simulink model "myfilterbank"  (Simulink 4.00)
settings: Solver=ode45  StartTime=0.0  StopTime=20000  RelTol=1e-3
libraries: ALTELINK x209, simulink_extras x2
settings Model: LastModifiedBy=Administrator

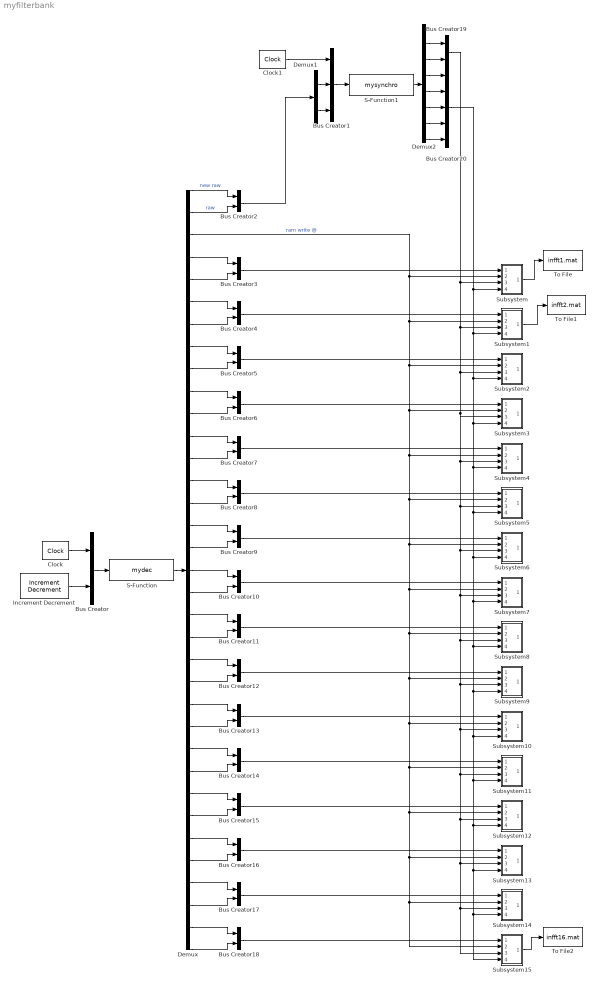
== system myfilterbank ==
  Bus Creator{,2..19} (19 alike) : BusCreator  Inputs=2
  Bus Creator1 : BusCreator  Inputs=3
  Bus Creator20 : BusCreator  Inputs=5
  Clock : simulink_extras/Flip Flops/Clock  MaskParam1=1
  Clock1 : simulink_extras/Flip Flops/Clock  MaskParam1=1
  Demux : Demux  Outputs=35  BusSelectionMode=off
  Demux1 : Demux  Outputs=2  BusSelectionMode=off
  Demux2 : Demux  Outputs=8  BusSelectionMode=off
  Increment Decrement : ALTELINK/Arithmetic/Increment Decrement  BusType=Unsigned Integer  bwl=20  bwr=0  direction=Increment  cst=1  clken=off  MaskValue=1
  S-Function : S-Function  FunctionName=mydec  Parameters=1,256,16,16  PortCounts=[]  SFunctionModules=''
  S-Function1 : S-Function  FunctionName=mysynchro  Parameters=1,256,16,16  PortCounts=[]  SFunctionModules=''
  Subsystem : Subsystem
      settings: RTWFcnNameOpts=Auto  RTWFileNameOpts=Auto
  Subsystem1 : Subsystem
      settings: RTWFcnNameOpts=Auto  RTWFileNameOpts=Auto
  Subsystem10 : Subsystem
      settings: RTWFcnNameOpts=Auto  RTWFileNameOpts=Auto
  Subsystem11 : Subsystem
      settings: RTWFcnNameOpts=Auto  RTWFileNameOpts=Auto
  Subsystem12 : Subsystem
      settings: RTWFcnNameOpts=Auto  RTWFileNameOpts=Auto
  Subsystem13 : Subsystem
      settings: RTWFcnNameOpts=Auto  RTWFileNameOpts=Auto
  Subsystem14 : Subsystem
      settings: RTWFcnNameOpts=Auto  RTWFileNameOpts=Auto
  Subsystem15 : Subsystem
      settings: RTWFcnNameOpts=Auto  RTWFileNameOpts=Auto
  Subsystem2 : Subsystem
      settings: RTWFcnNameOpts=Auto  RTWFileNameOpts=Auto
  Subsystem3 : Subsystem
      settings: RTWFcnNameOpts=Auto  RTWFileNameOpts=Auto
  Subsystem4 : Subsystem
      settings: RTWFcnNameOpts=Auto  RTWFileNameOpts=Auto
  Subsystem5 : Subsystem
      settings: RTWFcnNameOpts=Auto  RTWFileNameOpts=Auto
  Subsystem6 : Subsystem
      settings: RTWFcnNameOpts=Auto  RTWFileNameOpts=Auto
  Subsystem7 : Subsystem
      settings: RTWFcnNameOpts=Auto  RTWFileNameOpts=Auto
  Subsystem8 : Subsystem
      settings: RTWFcnNameOpts=Auto  RTWFileNameOpts=Auto
  Subsystem9 : Subsystem
      settings: RTWFcnNameOpts=Auto  RTWFileNameOpts=Auto
  To File : ToFile  Filename=infft1.mat  MatrixName=sig1  SampleTime=-1
  To File1 : ToFile  Filename=infft2.mat  MatrixName=sig2  SampleTime=-1
  To File2 : ToFile  Filename=infft16.mat  MatrixName=sig16  SampleTime=-1
  wires:
  S-Function/1 -> Demux/1
  Bus Creator/1 -> S-Function/1
  Clock/1 -> Bus Creator/1
  Increment Decrement/1 -> Bus Creator/2
  Demux/3 -> Subsystem/2(In2), Subsystem1/2(In2), Subsystem2/2(In2), Subsystem3/2(In2), Subsystem4/2(In2), Subsystem5/2(In2), Subsystem6/2(In2), Subsystem7/2(In2), Subsystem8/2(In2), Subsystem9/2(In2), Subsystem10/2(In2), Subsystem11/2(In2), Subsystem12/2(In2), Subsystem13/2(In2), Subsystem14/2(In2), Subsystem15/2(In2)  "ram write @"
  Clock1/1 -> Bus Creator1/1
  Bus Creator1/1 -> S-Function1/1
  Demux/1 -> Bus Creator2/1  "new raw"
  Demux/2 -> Bus Creator2/2  "raw"
  Bus Creator2/1 -> Demux1/1
  Demux1/1 -> Bus Creator1/2
  Demux1/2 -> Bus Creator1/3
  Demux/4 -> Bus Creator3/1
  Demux/5 -> Bus Creator3/2
  Bus Creator3/1 -> Subsystem/1(In1)
  Demux/6 -> Bus Creator4/1
  Demux/7 -> Bus Creator4/2
  Demux/8 -> Bus Creator5/1
  Demux/9 -> Bus Creator5/2
  Demux/10 -> Bus Creator6/1
  Demux/11 -> Bus Creator6/2
  Demux/12 -> Bus Creator7/1
  Demux/13 -> Bus Creator7/2
  Demux/14 -> Bus Creator8/1
  Demux/15 -> Bus Creator8/2
  Demux/16 -> Bus Creator9/1
  Demux/17 -> Bus Creator9/2
  Demux/18 -> Bus Creator10/1
  Demux/19 -> Bus Creator10/2
  Demux/20 -> Bus Creator11/1
  Demux/21 -> Bus Creator11/2
  Demux/22 -> Bus Creator12/1
  Demux/23 -> Bus Creator12/2
  Demux/24 -> Bus Creator13/1
  Demux/25 -> Bus Creator13/2
  Demux/26 -> Bus Creator14/1
  Demux/27 -> Bus Creator14/2
  Demux/28 -> Bus Creator15/1
  Demux/29 -> Bus Creator15/2
  Demux/30 -> Bus Creator16/1
  Demux/31 -> Bus Creator16/2
  Demux/32 -> Bus Creator17/1
  Demux/33 -> Bus Creator17/2
  Demux/34 -> Bus Creator18/1
  Demux/35 -> Bus Creator18/2
  Demux2/3 -> Bus Creator19/2
  Demux2/2 -> Bus Creator19/1
  Bus Creator19/1 -> Subsystem/3(In3), Subsystem1/3(In3), Subsystem2/3(In3), Subsystem3/3(In3), Subsystem4/3(In3), Subsystem5/3(In3), Subsystem6/3(In3), Subsystem7/3(In3), Subsystem8/3(In3), Subsystem9/3(In3), Subsystem10/3(In3), Subsystem11/3(In3), Subsystem12/3(In3), Subsystem13/3(In3), Subsystem14/3(In3), Subsystem15/3(In3)
  S-Function1/1 -> Demux2/1
  Demux2/4 -> Bus Creator20/1
  Demux2/5 -> Bus Creator20/2
  Demux2/6 -> Bus Creator20/3
  Demux2/7 -> Bus Creator20/4
  Demux2/8 -> Bus Creator20/5
  Bus Creator20/1 -> Subsystem/4(In4), Subsystem1/4(In4), Subsystem2/4(In4), Subsystem3/4(In4), Subsystem4/4(In4), Subsystem5/4(In4), Subsystem6/4(In4), Subsystem7/4(In4), Subsystem8/4(In4), Subsystem9/4(In4), Subsystem10/4(In4), Subsystem11/4(In4), Subsystem12/4(In4), Subsystem13/4(In4), Subsystem14/4(In4), Subsystem15/4(In4)
  Subsystem/1(Out1) -> To File/1
  Bus Creator4/1 -> Subsystem1/1(In1)
  Bus Creator5/1 -> Subsystem2/1(In1)
  Bus Creator6/1 -> Subsystem3/1(In1)
  Subsystem1/1(Out1) -> To File1/1
  Bus Creator7/1 -> Subsystem4/1(In1)
  Bus Creator8/1 -> Subsystem5/1(In1)
  Bus Creator9/1 -> Subsystem6/1(In1)
  Bus Creator10/1 -> Subsystem7/1(In1)
  Bus Creator11/1 -> Subsystem8/1(In1)
  Bus Creator12/1 -> Subsystem9/1(In1)
  Bus Creator13/1 -> Subsystem10/1(In1)
  Bus Creator14/1 -> Subsystem11/1(In1)
  Bus Creator15/1 -> Subsystem12/1(In1)
  Bus Creator16/1 -> Subsystem13/1(In1)
  Bus Creator17/1 -> Subsystem14/1(In1)
  Bus Creator18/1 -> Subsystem15/1(In1)
  Subsystem15/1(Out1) -> To File2/1

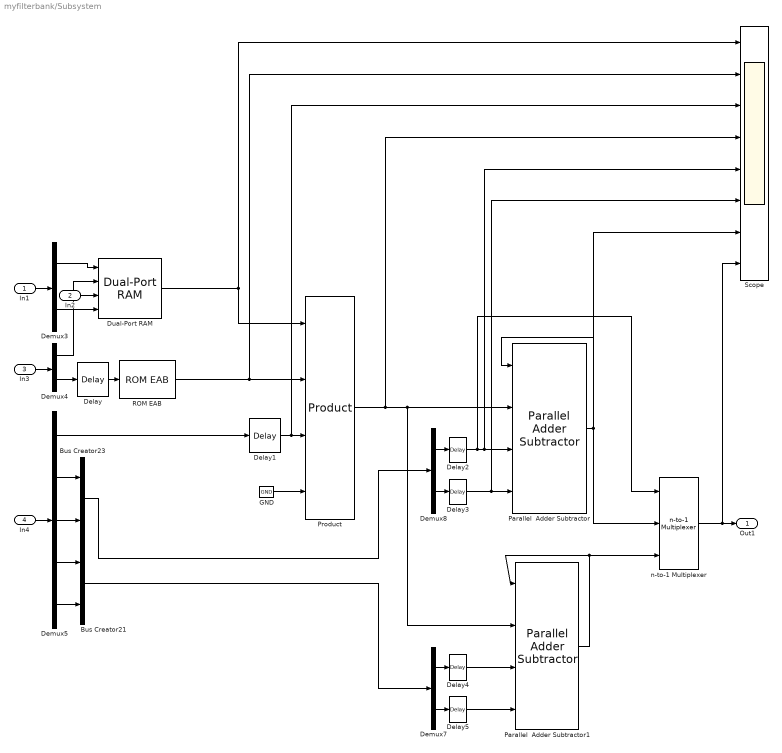
== system myfilterbank/Subsystem ==
  In1 : Inport  Port=1  LatchInput=off
  In2 : Inport  Port=2  LatchInput=off
  In3 : Inport  Port=3  LatchInput=off
  In4 : Inport  Port=4  LatchInput=off
  Bus Creator21 : BusCreator  Inputs=2
  Bus Creator23 : BusCreator  Inputs=2
  Delay : ALTELINK/Storage/Delay  depth=1  clken=off  MaskValue=1
  Delay1 : ALTELINK/Storage/Delay  depth=2  clken=off  MaskValue=1
  Delay{2..5} (4 alike) : ALTELINK/Storage/Delay  depth=3  clken=off  MaskValue=1
  Demux{3..4,7..8} (4 alike) : Demux  Outputs=2  BusSelectionMode=off
  Demux5 : Demux  Outputs=5  BusSelectionMode=off
  Dual-Port RAM : ALTELINK/Storage/Dual-Port RAM  bwaddr=9  MaskValue=1
  GND : ALTELINK/Bus Manipulation/GND
  Parallel  Adder Subtractor : ALTELINK/Arithmetic/Parallel  Adder Subtractor  Inputs=2  direction=++  pipeline=on  clken=on  MaskValue=1
  Parallel  Adder Subtractor1 : ALTELINK/Arithmetic/Parallel  Adder Subtractor  Inputs=2  direction=++  pipeline=on  clken=on  MaskValue=1
  Product : ALTELINK/Arithmetic/Product  pipeline=1  lpm=off  eab=off  clken=on  MaskValue=1
  ROM EAB : ALTELINK/Storage/ROM EAB  BusType=Signed Integer  bwl=14  bwr=0  bwaddr=8  Inputs=sub1.hex  MaskValue=1
  Scope : Scope  NumInputPorts=8
      settings: TimeRange=106.7708333333333  YMin=-5~-5~-5~-5~-5~0~-5~-5  YMax=5~5~5~5~5~1~5~5  SaveToWorkspace=off  SaveName=ScopeData  LimitDataPoints=on  MaxDataPoints=20000
  n-to-1 Multiplexer : ALTELINK/Gates/n-to-1 Multiplexer  Inputs=2  BusType=off
  Out1 : Outport  Port=1
  wires:
  Dual-Port RAM/1 -> Product/1, Scope/1
  ROM EAB/1 -> Product/2, Scope/2
  Product/1 -> Parallel  Adder Subtractor/2, Parallel  Adder Subtractor1/2, Scope/4
  Parallel  Adder Subtractor1/1 -> Parallel  Adder Subtractor1/1, n-to-1 Multiplexer/3
  Parallel  Adder Subtractor/1 -> Parallel  Adder Subtractor/1, Scope/7, n-to-1 Multiplexer/2
  Delay/1 -> ROM EAB/1
  GND/1 -> Product/4
  Demux3/2 -> Dual-Port RAM/4
  Demux3/1 -> Dual-Port RAM/1
  Demux4/1 -> Dual-Port RAM/2
  Demux4/2 -> Delay/1
  Demux5/1 -> Delay1/1
  Delay1/1 -> Product/3, Scope/3
  Demux7/2 -> Delay5/1
  Demux7/1 -> Delay4/1
  Demux8/2 -> Delay3/1
  Demux8/1 -> Delay2/1
  Demux5/5 -> Bus Creator21/2
  Demux5/4 -> Bus Creator21/1
  Demux5/3 -> Bus Creator23/2
  Demux5/2 -> Bus Creator23/1
  Bus Creator21/1 -> Demux7/1
  Bus Creator23/1 -> Demux8/1
  Delay2/1 -> n-to-1 Multiplexer/1, Parallel  Adder Subtractor/3, Scope/5
  Delay3/1 -> Parallel  Adder Subtractor/4, Scope/6
  Delay4/1 -> Parallel  Adder Subtractor1/3
  Delay5/1 -> Parallel  Adder Subtractor1/4
  n-to-1 Multiplexer/1 -> Scope/8, Out1/1
  In1/1 -> Demux3/1
  In2/1 -> Dual-Port RAM/3
  In3/1 -> Demux4/1
  In4/1 -> Demux5/1

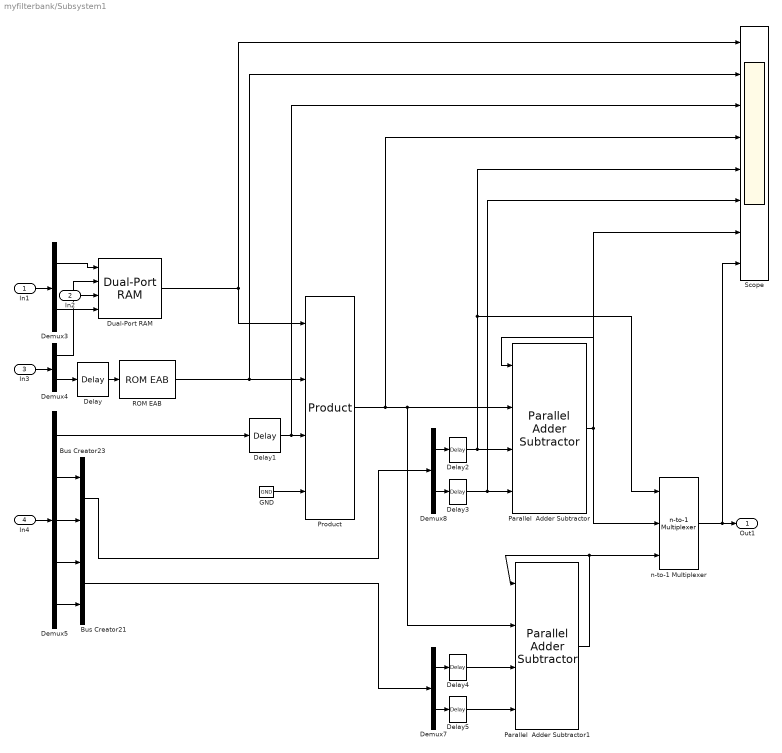
== system myfilterbank/Subsystem1 ==
  In1 : Inport  Port=1  LatchInput=off
  In2 : Inport  Port=2  LatchInput=off
  In3 : Inport  Port=3  LatchInput=off
  In4 : Inport  Port=4  LatchInput=off
  Bus Creator21 : BusCreator  Inputs=2
  Bus Creator23 : BusCreator  Inputs=2
  Delay : ALTELINK/Storage/Delay  depth=1  clken=off  MaskValue=1
  Delay1 : ALTELINK/Storage/Delay  depth=2  clken=off  MaskValue=1
  Delay{2..5} (4 alike) : ALTELINK/Storage/Delay  depth=3  clken=off  MaskValue=1
  Demux{3..4,7..8} (4 alike) : Demux  Outputs=2  BusSelectionMode=off
  Demux5 : Demux  Outputs=5  BusSelectionMode=off
  Dual-Port RAM : ALTELINK/Storage/Dual-Port RAM  bwaddr=9  MaskValue=1
  GND : ALTELINK/Bus Manipulation/GND
  Parallel  Adder Subtractor : ALTELINK/Arithmetic/Parallel  Adder Subtractor  Inputs=2  direction=++  pipeline=on  clken=on  MaskValue=1
  Parallel  Adder Subtractor1 : ALTELINK/Arithmetic/Parallel  Adder Subtractor  Inputs=2  direction=++  pipeline=on  clken=on  MaskValue=1
  Product : ALTELINK/Arithmetic/Product  pipeline=1  lpm=off  eab=off  clken=on  MaskValue=1
  ROM EAB : ALTELINK/Storage/ROM EAB  BusType=Signed Integer  bwl=14  bwr=0  bwaddr=9  Inputs=onlyone.hex  MaskValue=1
  Scope : Scope  NumInputPorts=8
      settings: TimeRange=auto  YMin=-5~-5~-5~-5~-5~-5~-5~-5  YMax=5~5~5~5~5~5~5~5  SaveToWorkspace=off  SaveName=ScopeData  LimitDataPoints=on  MaxDataPoints=20000
  n-to-1 Multiplexer : ALTELINK/Gates/n-to-1 Multiplexer  Inputs=2  BusType=off
  Out1 : Outport  Port=1
  wires:
  Dual-Port RAM/1 -> Product/1, Scope/1
  ROM EAB/1 -> Product/2, Scope/2
  Product/1 -> Parallel  Adder Subtractor/2, Parallel  Adder Subtractor1/2, Scope/4
  Parallel  Adder Subtractor1/1 -> Parallel  Adder Subtractor1/1, n-to-1 Multiplexer/3
  Parallel  Adder Subtractor/1 -> Parallel  Adder Subtractor/1, Scope/7, n-to-1 Multiplexer/2
  Delay/1 -> ROM EAB/1
  GND/1 -> Product/4
  Demux3/2 -> Dual-Port RAM/4
  Demux3/1 -> Dual-Port RAM/1
  Demux4/1 -> Dual-Port RAM/2
  Demux4/2 -> Delay/1
  Demux5/1 -> Delay1/1
  Delay1/1 -> Product/3, Scope/3
  Demux7/2 -> Delay5/1
  Demux7/1 -> Delay4/1
  Demux8/2 -> Delay3/1
  Demux8/1 -> Delay2/1
  Demux5/5 -> Bus Creator21/2
  Demux5/4 -> Bus Creator21/1
  Demux5/3 -> Bus Creator23/2
  Demux5/2 -> Bus Creator23/1
  Bus Creator21/1 -> Demux7/1
  Bus Creator23/1 -> Demux8/1
  Delay2/1 -> Parallel  Adder Subtractor/3, Scope/5, n-to-1 Multiplexer/1
  Delay3/1 -> Parallel  Adder Subtractor/4, Scope/6
  Delay4/1 -> Parallel  Adder Subtractor1/3
  Delay5/1 -> Parallel  Adder Subtractor1/4
  n-to-1 Multiplexer/1 -> Scope/8, Out1/1
  In1/1 -> Demux3/1
  In2/1 -> Dual-Port RAM/3
  In3/1 -> Demux4/1
  In4/1 -> Demux5/1

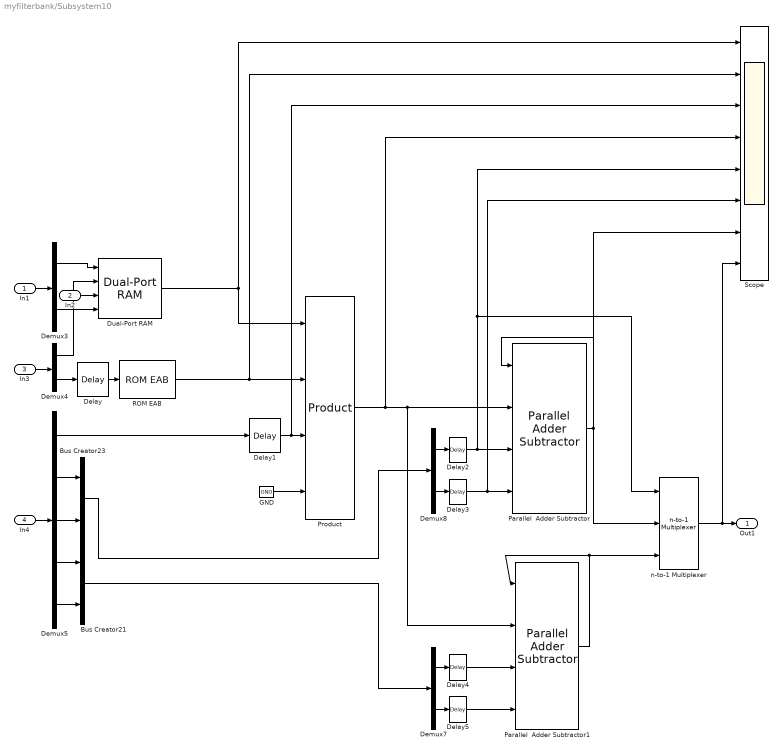
== system myfilterbank/Subsystem10 ==
  In1 : Inport  Port=1  LatchInput=off
  In2 : Inport  Port=2  LatchInput=off
  In3 : Inport  Port=3  LatchInput=off
  In4 : Inport  Port=4  LatchInput=off
  Bus Creator21 : BusCreator  Inputs=2
  Bus Creator23 : BusCreator  Inputs=2
  Delay : ALTELINK/Storage/Delay  depth=1  clken=off  MaskValue=1
  Delay1 : ALTELINK/Storage/Delay  depth=2  clken=off  MaskValue=1
  Delay{2..5} (4 alike) : ALTELINK/Storage/Delay  depth=3  clken=off  MaskValue=1
  Demux{3..4,7..8} (4 alike) : Demux  Outputs=2  BusSelectionMode=off
  Demux5 : Demux  Outputs=5  BusSelectionMode=off
  Dual-Port RAM : ALTELINK/Storage/Dual-Port RAM  bwaddr=9  MaskValue=1
  GND : ALTELINK/Bus Manipulation/GND
  Parallel  Adder Subtractor : ALTELINK/Arithmetic/Parallel  Adder Subtractor  Inputs=2  direction=++  pipeline=on  clken=on  MaskValue=1
  Parallel  Adder Subtractor1 : ALTELINK/Arithmetic/Parallel  Adder Subtractor  Inputs=2  direction=++  pipeline=on  clken=on  MaskValue=1
  Product : ALTELINK/Arithmetic/Product  pipeline=1  lpm=off  eab=off  clken=on  MaskValue=1
  ROM EAB : ALTELINK/Storage/ROM EAB  BusType=Signed Integer  bwl=14  bwr=0  bwaddr=9  Inputs=onlyone.hex  MaskValue=1
  Scope : Scope  NumInputPorts=8
      settings: TimeRange=auto  YMin=-5~-5~-5~-5~-5~-5~-5~-5  YMax=5~5~5~5~5~5~5~5  SaveToWorkspace=off  SaveName=ScopeData  LimitDataPoints=on  MaxDataPoints=20000
  n-to-1 Multiplexer : ALTELINK/Gates/n-to-1 Multiplexer  Inputs=2  BusType=off
  Out1 : Outport  Port=1
  wires:
  Dual-Port RAM/1 -> Product/1, Scope/1
  ROM EAB/1 -> Product/2, Scope/2
  Product/1 -> Parallel  Adder Subtractor/2, Parallel  Adder Subtractor1/2, Scope/4
  Parallel  Adder Subtractor1/1 -> Parallel  Adder Subtractor1/1, n-to-1 Multiplexer/3
  Parallel  Adder Subtractor/1 -> Parallel  Adder Subtractor/1, Scope/7, n-to-1 Multiplexer/2
  Delay/1 -> ROM EAB/1
  GND/1 -> Product/4
  Demux3/2 -> Dual-Port RAM/4
  Demux3/1 -> Dual-Port RAM/1
  Demux4/1 -> Dual-Port RAM/2
  Demux4/2 -> Delay/1
  Demux5/1 -> Delay1/1
  Delay1/1 -> Product/3, Scope/3
  Demux7/2 -> Delay5/1
  Demux7/1 -> Delay4/1
  Demux8/2 -> Delay3/1
  Demux8/1 -> Delay2/1
  Demux5/5 -> Bus Creator21/2
  Demux5/4 -> Bus Creator21/1
  Demux5/3 -> Bus Creator23/2
  Demux5/2 -> Bus Creator23/1
  Bus Creator21/1 -> Demux7/1
  Bus Creator23/1 -> Demux8/1
  Delay2/1 -> Parallel  Adder Subtractor/3, Scope/5, n-to-1 Multiplexer/1
  Delay3/1 -> Parallel  Adder Subtractor/4, Scope/6
  Delay4/1 -> Parallel  Adder Subtractor1/3
  Delay5/1 -> Parallel  Adder Subtractor1/4
  n-to-1 Multiplexer/1 -> Scope/8, Out1/1
  In1/1 -> Demux3/1
  In2/1 -> Dual-Port RAM/3
  In3/1 -> Demux4/1
  In4/1 -> Demux5/1

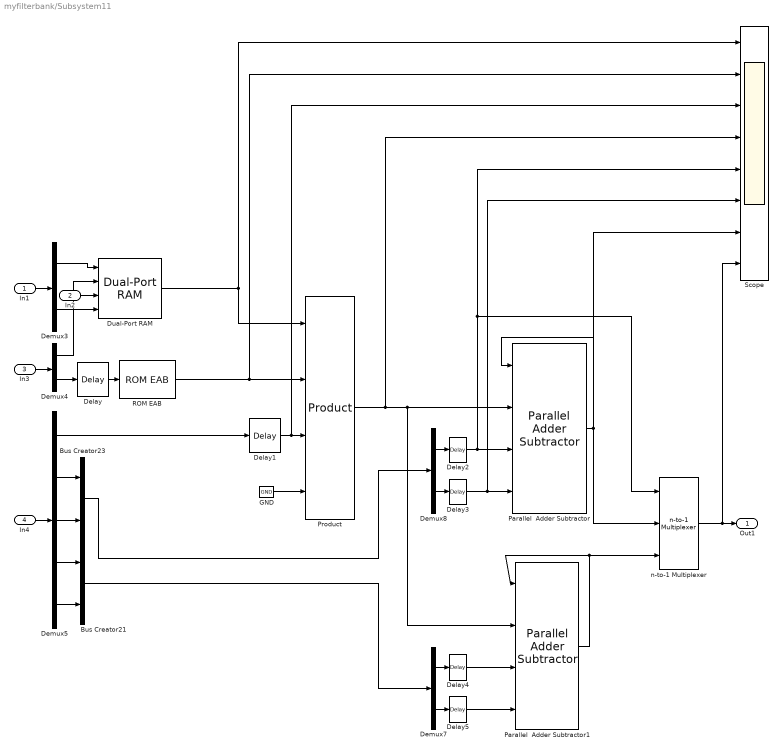
== system myfilterbank/Subsystem11 ==
  In1 : Inport  Port=1  LatchInput=off
  In2 : Inport  Port=2  LatchInput=off
  In3 : Inport  Port=3  LatchInput=off
  In4 : Inport  Port=4  LatchInput=off
  Bus Creator21 : BusCreator  Inputs=2
  Bus Creator23 : BusCreator  Inputs=2
  Delay : ALTELINK/Storage/Delay  depth=1  clken=off  MaskValue=1
  Delay1 : ALTELINK/Storage/Delay  depth=2  clken=off  MaskValue=1
  Delay{2..5} (4 alike) : ALTELINK/Storage/Delay  depth=3  clken=off  MaskValue=1
  Demux{3..4,7..8} (4 alike) : Demux  Outputs=2  BusSelectionMode=off
  Demux5 : Demux  Outputs=5  BusSelectionMode=off
  Dual-Port RAM : ALTELINK/Storage/Dual-Port RAM  bwaddr=9  MaskValue=1
  GND : ALTELINK/Bus Manipulation/GND
  Parallel  Adder Subtractor : ALTELINK/Arithmetic/Parallel  Adder Subtractor  Inputs=2  direction=++  pipeline=on  clken=on  MaskValue=1
  Parallel  Adder Subtractor1 : ALTELINK/Arithmetic/Parallel  Adder Subtractor  Inputs=2  direction=++  pipeline=on  clken=on  MaskValue=1
  Product : ALTELINK/Arithmetic/Product  pipeline=1  lpm=off  eab=off  clken=on  MaskValue=1
  ROM EAB : ALTELINK/Storage/ROM EAB  BusType=Signed Integer  bwl=14  bwr=0  bwaddr=9  Inputs=onlyone.hex  MaskValue=1
  Scope : Scope  NumInputPorts=8
      settings: TimeRange=auto  YMin=-5~-5~-5~-5~-5~-5~-5~-5  YMax=5~5~5~5~5~5~5~5  SaveToWorkspace=off  SaveName=ScopeData  LimitDataPoints=on  MaxDataPoints=20000
  n-to-1 Multiplexer : ALTELINK/Gates/n-to-1 Multiplexer  Inputs=2  BusType=off
  Out1 : Outport  Port=1
  wires:
  Dual-Port RAM/1 -> Product/1, Scope/1
  ROM EAB/1 -> Product/2, Scope/2
  Product/1 -> Parallel  Adder Subtractor/2, Parallel  Adder Subtractor1/2, Scope/4
  Parallel  Adder Subtractor1/1 -> Parallel  Adder Subtractor1/1, n-to-1 Multiplexer/3
  Parallel  Adder Subtractor/1 -> Parallel  Adder Subtractor/1, Scope/7, n-to-1 Multiplexer/2
  Delay/1 -> ROM EAB/1
  GND/1 -> Product/4
  Demux3/2 -> Dual-Port RAM/4
  Demux3/1 -> Dual-Port RAM/1
  Demux4/1 -> Dual-Port RAM/2
  Demux4/2 -> Delay/1
  Demux5/1 -> Delay1/1
  Delay1/1 -> Product/3, Scope/3
  Demux7/2 -> Delay5/1
  Demux7/1 -> Delay4/1
  Demux8/2 -> Delay3/1
  Demux8/1 -> Delay2/1
  Demux5/5 -> Bus Creator21/2
  Demux5/4 -> Bus Creator21/1
  Demux5/3 -> Bus Creator23/2
  Demux5/2 -> Bus Creator23/1
  Bus Creator21/1 -> Demux7/1
  Bus Creator23/1 -> Demux8/1
  Delay2/1 -> Parallel  Adder Subtractor/3, Scope/5, n-to-1 Multiplexer/1
  Delay3/1 -> Parallel  Adder Subtractor/4, Scope/6
  Delay4/1 -> Parallel  Adder Subtractor1/3
  Delay5/1 -> Parallel  Adder Subtractor1/4
  n-to-1 Multiplexer/1 -> Scope/8, Out1/1
  In1/1 -> Demux3/1
  In2/1 -> Dual-Port RAM/3
  In3/1 -> Demux4/1
  In4/1 -> Demux5/1

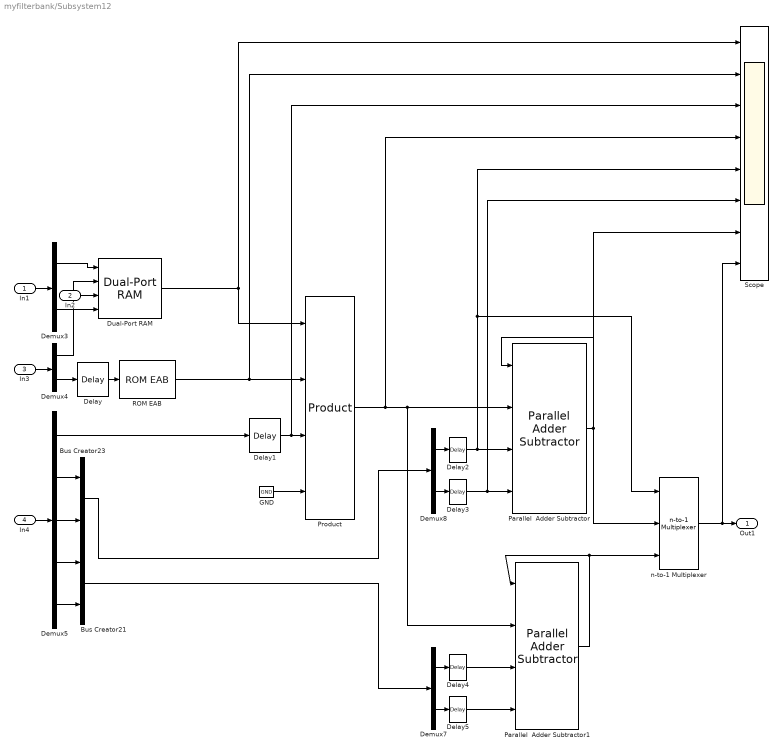
== system myfilterbank/Subsystem12 ==
  In1 : Inport  Port=1  LatchInput=off
  In2 : Inport  Port=2  LatchInput=off
  In3 : Inport  Port=3  LatchInput=off
  In4 : Inport  Port=4  LatchInput=off
  Bus Creator21 : BusCreator  Inputs=2
  Bus Creator23 : BusCreator  Inputs=2
  Delay : ALTELINK/Storage/Delay  depth=1  clken=off  MaskValue=1
  Delay1 : ALTELINK/Storage/Delay  depth=2  clken=off  MaskValue=1
  Delay{2..5} (4 alike) : ALTELINK/Storage/Delay  depth=3  clken=off  MaskValue=1
  Demux{3..4,7..8} (4 alike) : Demux  Outputs=2  BusSelectionMode=off
  Demux5 : Demux  Outputs=5  BusSelectionMode=off
  Dual-Port RAM : ALTELINK/Storage/Dual-Port RAM  bwaddr=9  MaskValue=1
  GND : ALTELINK/Bus Manipulation/GND
  Parallel  Adder Subtractor : ALTELINK/Arithmetic/Parallel  Adder Subtractor  Inputs=2  direction=++  pipeline=on  clken=on  MaskValue=1
  Parallel  Adder Subtractor1 : ALTELINK/Arithmetic/Parallel  Adder Subtractor  Inputs=2  direction=++  pipeline=on  clken=on  MaskValue=1
  Product : ALTELINK/Arithmetic/Product  pipeline=1  lpm=off  eab=off  clken=on  MaskValue=1
  ROM EAB : ALTELINK/Storage/ROM EAB  BusType=Signed Integer  bwl=14  bwr=0  bwaddr=9  Inputs=onlyone.hex  MaskValue=1
  Scope : Scope  NumInputPorts=8
      settings: TimeRange=auto  YMin=-5~-5~-5~-5~-5~-5~-5~-5  YMax=5~5~5~5~5~5~5~5  SaveToWorkspace=off  SaveName=ScopeData  LimitDataPoints=on  MaxDataPoints=20000
  n-to-1 Multiplexer : ALTELINK/Gates/n-to-1 Multiplexer  Inputs=2  BusType=off
  Out1 : Outport  Port=1
  wires:
  Dual-Port RAM/1 -> Product/1, Scope/1
  ROM EAB/1 -> Product/2, Scope/2
  Product/1 -> Parallel  Adder Subtractor/2, Parallel  Adder Subtractor1/2, Scope/4
  Parallel  Adder Subtractor1/1 -> Parallel  Adder Subtractor1/1, n-to-1 Multiplexer/3
  Parallel  Adder Subtractor/1 -> Parallel  Adder Subtractor/1, Scope/7, n-to-1 Multiplexer/2
  Delay/1 -> ROM EAB/1
  GND/1 -> Product/4
  Demux3/2 -> Dual-Port RAM/4
  Demux3/1 -> Dual-Port RAM/1
  Demux4/1 -> Dual-Port RAM/2
  Demux4/2 -> Delay/1
  Demux5/1 -> Delay1/1
  Delay1/1 -> Product/3, Scope/3
  Demux7/2 -> Delay5/1
  Demux7/1 -> Delay4/1
  Demux8/2 -> Delay3/1
  Demux8/1 -> Delay2/1
  Demux5/5 -> Bus Creator21/2
  Demux5/4 -> Bus Creator21/1
  Demux5/3 -> Bus Creator23/2
  Demux5/2 -> Bus Creator23/1
  Bus Creator21/1 -> Demux7/1
  Bus Creator23/1 -> Demux8/1
  Delay2/1 -> Parallel  Adder Subtractor/3, Scope/5, n-to-1 Multiplexer/1
  Delay3/1 -> Parallel  Adder Subtractor/4, Scope/6
  Delay4/1 -> Parallel  Adder Subtractor1/3
  Delay5/1 -> Parallel  Adder Subtractor1/4
  n-to-1 Multiplexer/1 -> Scope/8, Out1/1
  In1/1 -> Demux3/1
  In2/1 -> Dual-Port RAM/3
  In3/1 -> Demux4/1
  In4/1 -> Demux5/1

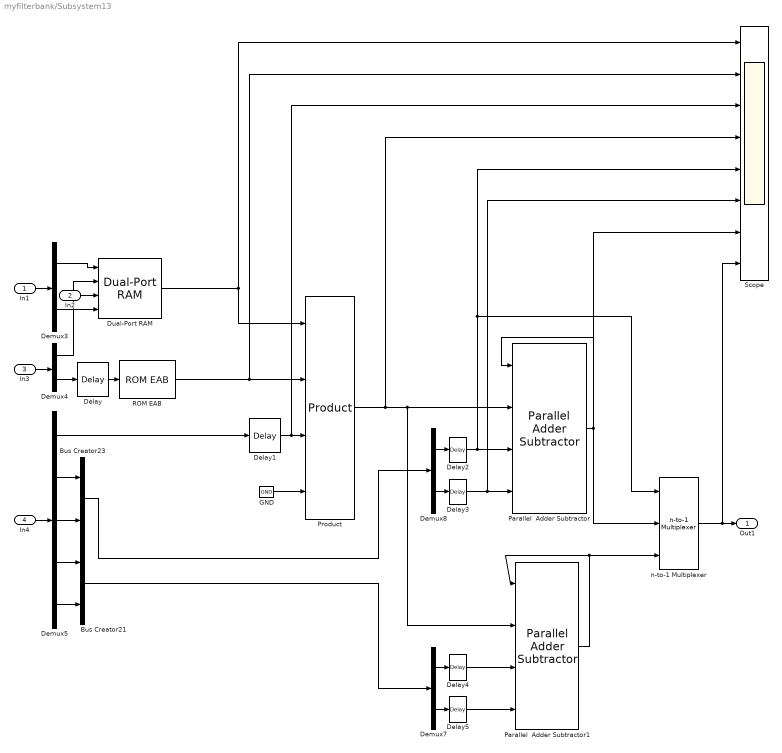
== system myfilterbank/Subsystem13 ==
  In1 : Inport  Port=1  LatchInput=off
  In2 : Inport  Port=2  LatchInput=off
  In3 : Inport  Port=3  LatchInput=off
  In4 : Inport  Port=4  LatchInput=off
  Bus Creator21 : BusCreator  Inputs=2
  Bus Creator23 : BusCreator  Inputs=2
  Delay : ALTELINK/Storage/Delay  depth=1  clken=off  MaskValue=1
  Delay1 : ALTELINK/Storage/Delay  depth=2  clken=off  MaskValue=1
  Delay{2..5} (4 alike) : ALTELINK/Storage/Delay  depth=3  clken=off  MaskValue=1
  Demux{3..4,7..8} (4 alike) : Demux  Outputs=2  BusSelectionMode=off
  Demux5 : Demux  Outputs=5  BusSelectionMode=off
  Dual-Port RAM : ALTELINK/Storage/Dual-Port RAM  bwaddr=9  MaskValue=1
  GND : ALTELINK/Bus Manipulation/GND
  Parallel  Adder Subtractor : ALTELINK/Arithmetic/Parallel  Adder Subtractor  Inputs=2  direction=++  pipeline=on  clken=on  MaskValue=1
  Parallel  Adder Subtractor1 : ALTELINK/Arithmetic/Parallel  Adder Subtractor  Inputs=2  direction=++  pipeline=on  clken=on  MaskValue=1
  Product : ALTELINK/Arithmetic/Product  pipeline=1  lpm=off  eab=off  clken=on  MaskValue=1
  ROM EAB : ALTELINK/Storage/ROM EAB  BusType=Signed Integer  bwl=14  bwr=0  bwaddr=9  Inputs=onlyone.hex  MaskValue=1
  Scope : Scope  NumInputPorts=8
      settings: TimeRange=auto  YMin=-5~-5~-5~-5~-5~-5~-5~-5  YMax=5~5~5~5~5~5~5~5  SaveToWorkspace=off  SaveName=ScopeData  LimitDataPoints=on  MaxDataPoints=20000
  n-to-1 Multiplexer : ALTELINK/Gates/n-to-1 Multiplexer  Inputs=2  BusType=off
  Out1 : Outport  Port=1
  wires:
  Dual-Port RAM/1 -> Product/1, Scope/1
  ROM EAB/1 -> Product/2, Scope/2
  Product/1 -> Parallel  Adder Subtractor/2, Parallel  Adder Subtractor1/2, Scope/4
  Parallel  Adder Subtractor1/1 -> Parallel  Adder Subtractor1/1, n-to-1 Multiplexer/3
  Parallel  Adder Subtractor/1 -> Parallel  Adder Subtractor/1, Scope/7, n-to-1 Multiplexer/2
  Delay/1 -> ROM EAB/1
  GND/1 -> Product/4
  Demux3/2 -> Dual-Port RAM/4
  Demux3/1 -> Dual-Port RAM/1
  Demux4/1 -> Dual-Port RAM/2
  Demux4/2 -> Delay/1
  Demux5/1 -> Delay1/1
  Delay1/1 -> Product/3, Scope/3
  Demux7/2 -> Delay5/1
  Demux7/1 -> Delay4/1
  Demux8/2 -> Delay3/1
  Demux8/1 -> Delay2/1
  Demux5/5 -> Bus Creator21/2
  Demux5/4 -> Bus Creator21/1
  Demux5/3 -> Bus Creator23/2
  Demux5/2 -> Bus Creator23/1
  Bus Creator21/1 -> Demux7/1
  Bus Creator23/1 -> Demux8/1
  Delay2/1 -> Parallel  Adder Subtractor/3, Scope/5, n-to-1 Multiplexer/1
  Delay3/1 -> Parallel  Adder Subtractor/4, Scope/6
  Delay4/1 -> Parallel  Adder Subtractor1/3
  Delay5/1 -> Parallel  Adder Subtractor1/4
  n-to-1 Multiplexer/1 -> Scope/8, Out1/1
  In1/1 -> Demux3/1
  In2/1 -> Dual-Port RAM/3
  In3/1 -> Demux4/1
  In4/1 -> Demux5/1

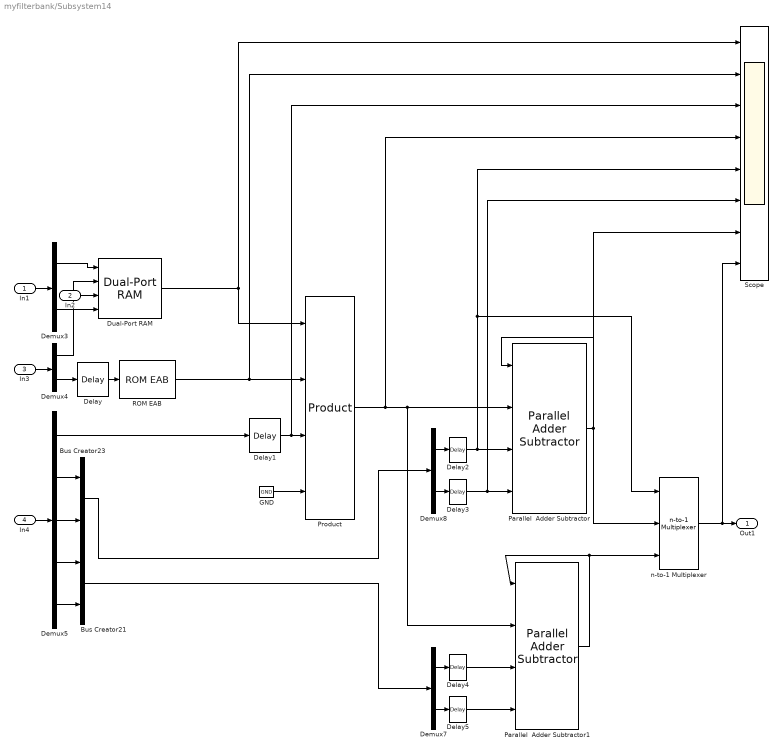
== system myfilterbank/Subsystem14 ==
  In1 : Inport  Port=1  LatchInput=off
  In2 : Inport  Port=2  LatchInput=off
  In3 : Inport  Port=3  LatchInput=off
  In4 : Inport  Port=4  LatchInput=off
  Bus Creator21 : BusCreator  Inputs=2
  Bus Creator23 : BusCreator  Inputs=2
  Delay : ALTELINK/Storage/Delay  depth=1  clken=off  MaskValue=1
  Delay1 : ALTELINK/Storage/Delay  depth=2  clken=off  MaskValue=1
  Delay{2..5} (4 alike) : ALTELINK/Storage/Delay  depth=3  clken=off  MaskValue=1
  Demux{3..4,7..8} (4 alike) : Demux  Outputs=2  BusSelectionMode=off
  Demux5 : Demux  Outputs=5  BusSelectionMode=off
  Dual-Port RAM : ALTELINK/Storage/Dual-Port RAM  bwaddr=9  MaskValue=1
  GND : ALTELINK/Bus Manipulation/GND
  Parallel  Adder Subtractor : ALTELINK/Arithmetic/Parallel  Adder Subtractor  Inputs=2  direction=++  pipeline=on  clken=on  MaskValue=1
  Parallel  Adder Subtractor1 : ALTELINK/Arithmetic/Parallel  Adder Subtractor  Inputs=2  direction=++  pipeline=on  clken=on  MaskValue=1
  Product : ALTELINK/Arithmetic/Product  pipeline=1  lpm=off  eab=off  clken=on  MaskValue=1
  ROM EAB : ALTELINK/Storage/ROM EAB  BusType=Signed Integer  bwl=14  bwr=0  bwaddr=9  Inputs=onlyone.hex  MaskValue=1
  Scope : Scope  NumInputPorts=8
      settings: TimeRange=auto  YMin=-5~-5~-5~-5~-5~-5~-5~-5  YMax=5~5~5~5~5~5~5~5  SaveToWorkspace=off  SaveName=ScopeData  LimitDataPoints=on  MaxDataPoints=20000
  n-to-1 Multiplexer : ALTELINK/Gates/n-to-1 Multiplexer  Inputs=2  BusType=off
  Out1 : Outport  Port=1
  wires:
  Dual-Port RAM/1 -> Product/1, Scope/1
  ROM EAB/1 -> Product/2, Scope/2
  Product/1 -> Parallel  Adder Subtractor/2, Parallel  Adder Subtractor1/2, Scope/4
  Parallel  Adder Subtractor1/1 -> Parallel  Adder Subtractor1/1, n-to-1 Multiplexer/3
  Parallel  Adder Subtractor/1 -> Parallel  Adder Subtractor/1, Scope/7, n-to-1 Multiplexer/2
  Delay/1 -> ROM EAB/1
  GND/1 -> Product/4
  Demux3/2 -> Dual-Port RAM/4
  Demux3/1 -> Dual-Port RAM/1
  Demux4/1 -> Dual-Port RAM/2
  Demux4/2 -> Delay/1
  Demux5/1 -> Delay1/1
  Delay1/1 -> Product/3, Scope/3
  Demux7/2 -> Delay5/1
  Demux7/1 -> Delay4/1
  Demux8/2 -> Delay3/1
  Demux8/1 -> Delay2/1
  Demux5/5 -> Bus Creator21/2
  Demux5/4 -> Bus Creator21/1
  Demux5/3 -> Bus Creator23/2
  Demux5/2 -> Bus Creator23/1
  Bus Creator21/1 -> Demux7/1
  Bus Creator23/1 -> Demux8/1
  Delay2/1 -> Parallel  Adder Subtractor/3, Scope/5, n-to-1 Multiplexer/1
  Delay3/1 -> Parallel  Adder Subtractor/4, Scope/6
  Delay4/1 -> Parallel  Adder Subtractor1/3
  Delay5/1 -> Parallel  Adder Subtractor1/4
  n-to-1 Multiplexer/1 -> Scope/8, Out1/1
  In1/1 -> Demux3/1
  In2/1 -> Dual-Port RAM/3
  In3/1 -> Demux4/1
  In4/1 -> Demux5/1

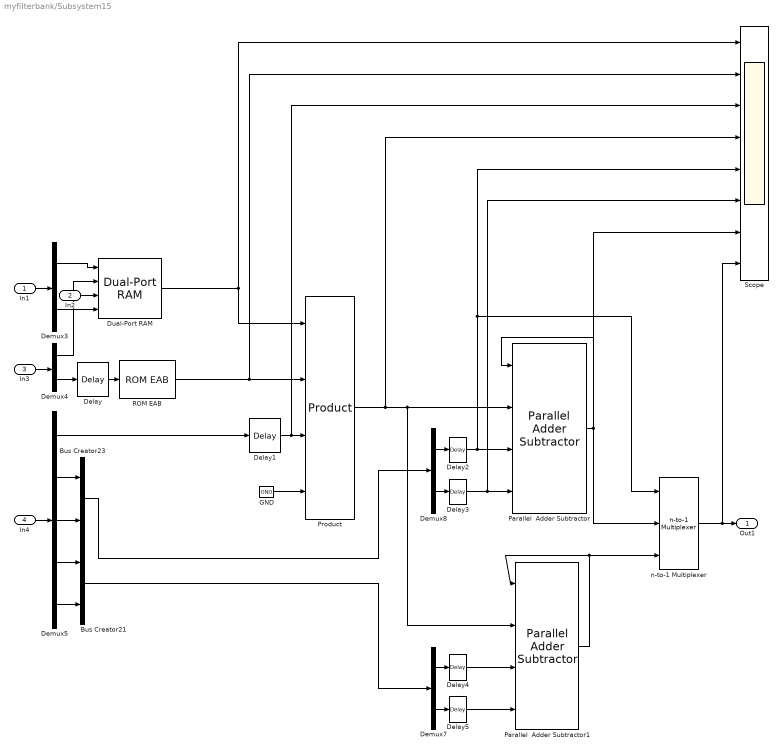
== system myfilterbank/Subsystem15 ==
  In1 : Inport  Port=1  LatchInput=off
  In2 : Inport  Port=2  LatchInput=off
  In3 : Inport  Port=3  LatchInput=off
  In4 : Inport  Port=4  LatchInput=off
  Bus Creator21 : BusCreator  Inputs=2
  Bus Creator23 : BusCreator  Inputs=2
  Delay : ALTELINK/Storage/Delay  depth=1  clken=off  MaskValue=1
  Delay1 : ALTELINK/Storage/Delay  depth=2  clken=off  MaskValue=1
  Delay{2..5} (4 alike) : ALTELINK/Storage/Delay  depth=3  clken=off  MaskValue=1
  Demux{3..4,7..8} (4 alike) : Demux  Outputs=2  BusSelectionMode=off
  Demux5 : Demux  Outputs=5  BusSelectionMode=off
  Dual-Port RAM : ALTELINK/Storage/Dual-Port RAM  bwaddr=9  MaskValue=1
  GND : ALTELINK/Bus Manipulation/GND
  Parallel  Adder Subtractor : ALTELINK/Arithmetic/Parallel  Adder Subtractor  Inputs=2  direction=++  pipeline=on  clken=on  MaskValue=1
  Parallel  Adder Subtractor1 : ALTELINK/Arithmetic/Parallel  Adder Subtractor  Inputs=2  direction=++  pipeline=on  clken=on  MaskValue=1
  Product : ALTELINK/Arithmetic/Product  pipeline=1  lpm=off  eab=off  clken=on  MaskValue=1
  ROM EAB : ALTELINK/Storage/ROM EAB  BusType=Signed Integer  bwl=14  bwr=0  bwaddr=9  Inputs=onlyone.hex  MaskValue=1
  Scope : Scope  NumInputPorts=8
      settings: TimeRange=auto  YMin=-5~-5~-5~-5~-5~-5~-5~-5  YMax=5~5~5~5~5~5~5~5  SaveToWorkspace=off  SaveName=ScopeData  LimitDataPoints=on  MaxDataPoints=20000
  n-to-1 Multiplexer : ALTELINK/Gates/n-to-1 Multiplexer  Inputs=2  BusType=off
  Out1 : Outport  Port=1
  wires:
  Dual-Port RAM/1 -> Product/1, Scope/1
  ROM EAB/1 -> Product/2, Scope/2
  Product/1 -> Parallel  Adder Subtractor/2, Parallel  Adder Subtractor1/2, Scope/4
  Parallel  Adder Subtractor1/1 -> Parallel  Adder Subtractor1/1, n-to-1 Multiplexer/3
  Parallel  Adder Subtractor/1 -> Parallel  Adder Subtractor/1, Scope/7, n-to-1 Multiplexer/2
  Delay/1 -> ROM EAB/1
  GND/1 -> Product/4
  Demux3/2 -> Dual-Port RAM/4
  Demux3/1 -> Dual-Port RAM/1
  Demux4/1 -> Dual-Port RAM/2
  Demux4/2 -> Delay/1
  Demux5/1 -> Delay1/1
  Delay1/1 -> Product/3, Scope/3
  Demux7/2 -> Delay5/1
  Demux7/1 -> Delay4/1
  Demux8/2 -> Delay3/1
  Demux8/1 -> Delay2/1
  Demux5/5 -> Bus Creator21/2
  Demux5/4 -> Bus Creator21/1
  Demux5/3 -> Bus Creator23/2
  Demux5/2 -> Bus Creator23/1
  Bus Creator21/1 -> Demux7/1
  Bus Creator23/1 -> Demux8/1
  Delay2/1 -> Parallel  Adder Subtractor/3, Scope/5, n-to-1 Multiplexer/1
  Delay3/1 -> Parallel  Adder Subtractor/4, Scope/6
  Delay4/1 -> Parallel  Adder Subtractor1/3
  Delay5/1 -> Parallel  Adder Subtractor1/4
  n-to-1 Multiplexer/1 -> Scope/8, Out1/1
  In1/1 -> Demux3/1
  In2/1 -> Dual-Port RAM/3
  In3/1 -> Demux4/1
  In4/1 -> Demux5/1

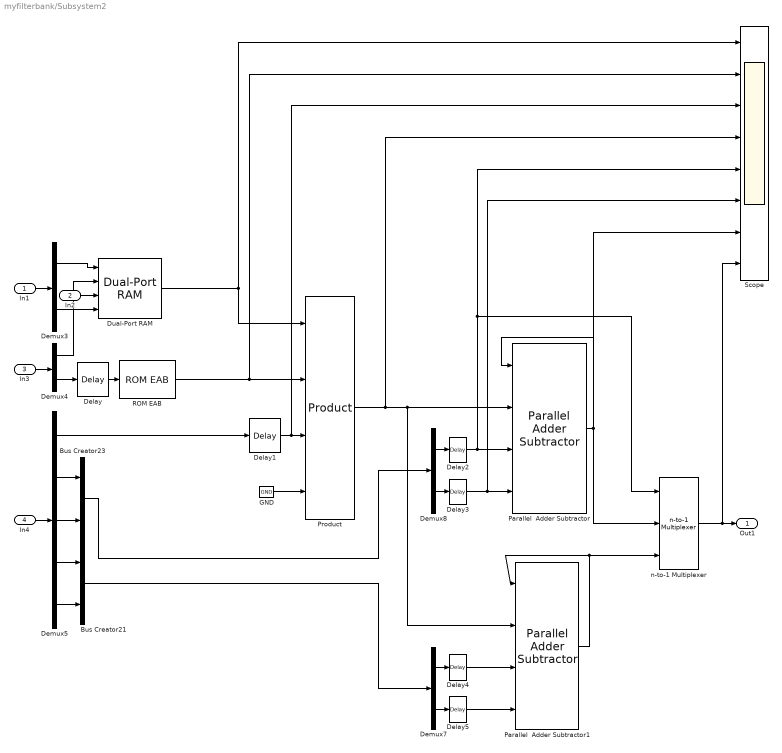
== system myfilterbank/Subsystem2 ==
  In1 : Inport  Port=1  LatchInput=off
  In2 : Inport  Port=2  LatchInput=off
  In3 : Inport  Port=3  LatchInput=off
  In4 : Inport  Port=4  LatchInput=off
  Bus Creator21 : BusCreator  Inputs=2
  Bus Creator23 : BusCreator  Inputs=2
  Delay : ALTELINK/Storage/Delay  depth=1  clken=off  MaskValue=1
  Delay1 : ALTELINK/Storage/Delay  depth=2  clken=off  MaskValue=1
  Delay{2..5} (4 alike) : ALTELINK/Storage/Delay  depth=3  clken=off  MaskValue=1
  Demux{3..4,7..8} (4 alike) : Demux  Outputs=2  BusSelectionMode=off
  Demux5 : Demux  Outputs=5  BusSelectionMode=off
  Dual-Port RAM : ALTELINK/Storage/Dual-Port RAM  bwaddr=9  MaskValue=1
  GND : ALTELINK/Bus Manipulation/GND
  Parallel  Adder Subtractor : ALTELINK/Arithmetic/Parallel  Adder Subtractor  Inputs=2  direction=++  pipeline=on  clken=on  MaskValue=1
  Parallel  Adder Subtractor1 : ALTELINK/Arithmetic/Parallel  Adder Subtractor  Inputs=2  direction=++  pipeline=on  clken=on  MaskValue=1
  Product : ALTELINK/Arithmetic/Product  pipeline=1  lpm=off  eab=off  clken=on  MaskValue=1
  ROM EAB : ALTELINK/Storage/ROM EAB  BusType=Signed Integer  bwl=14  bwr=0  bwaddr=9  Inputs=onlyone.hex  MaskValue=1
  Scope : Scope  NumInputPorts=8
      settings: TimeRange=auto  YMin=-5~-5~-5~-5~-5~-5~-5~-5  YMax=5~5~5~5~5~5~5~5  SaveToWorkspace=off  SaveName=ScopeData  LimitDataPoints=on  MaxDataPoints=20000
  n-to-1 Multiplexer : ALTELINK/Gates/n-to-1 Multiplexer  Inputs=2  BusType=off
  Out1 : Outport  Port=1
  wires:
  Dual-Port RAM/1 -> Product/1, Scope/1
  ROM EAB/1 -> Product/2, Scope/2
  Product/1 -> Parallel  Adder Subtractor/2, Parallel  Adder Subtractor1/2, Scope/4
  Parallel  Adder Subtractor1/1 -> Parallel  Adder Subtractor1/1, n-to-1 Multiplexer/3
  Parallel  Adder Subtractor/1 -> Parallel  Adder Subtractor/1, Scope/7, n-to-1 Multiplexer/2
  Delay/1 -> ROM EAB/1
  GND/1 -> Product/4
  Demux3/2 -> Dual-Port RAM/4
  Demux3/1 -> Dual-Port RAM/1
  Demux4/1 -> Dual-Port RAM/2
  Demux4/2 -> Delay/1
  Demux5/1 -> Delay1/1
  Delay1/1 -> Product/3, Scope/3
  Demux7/2 -> Delay5/1
  Demux7/1 -> Delay4/1
  Demux8/2 -> Delay3/1
  Demux8/1 -> Delay2/1
  Demux5/5 -> Bus Creator21/2
  Demux5/4 -> Bus Creator21/1
  Demux5/3 -> Bus Creator23/2
  Demux5/2 -> Bus Creator23/1
  Bus Creator21/1 -> Demux7/1
  Bus Creator23/1 -> Demux8/1
  Delay2/1 -> Parallel  Adder Subtractor/3, Scope/5, n-to-1 Multiplexer/1
  Delay3/1 -> Parallel  Adder Subtractor/4, Scope/6
  Delay4/1 -> Parallel  Adder Subtractor1/3
  Delay5/1 -> Parallel  Adder Subtractor1/4
  n-to-1 Multiplexer/1 -> Scope/8, Out1/1
  In1/1 -> Demux3/1
  In2/1 -> Dual-Port RAM/3
  In3/1 -> Demux4/1
  In4/1 -> Demux5/1

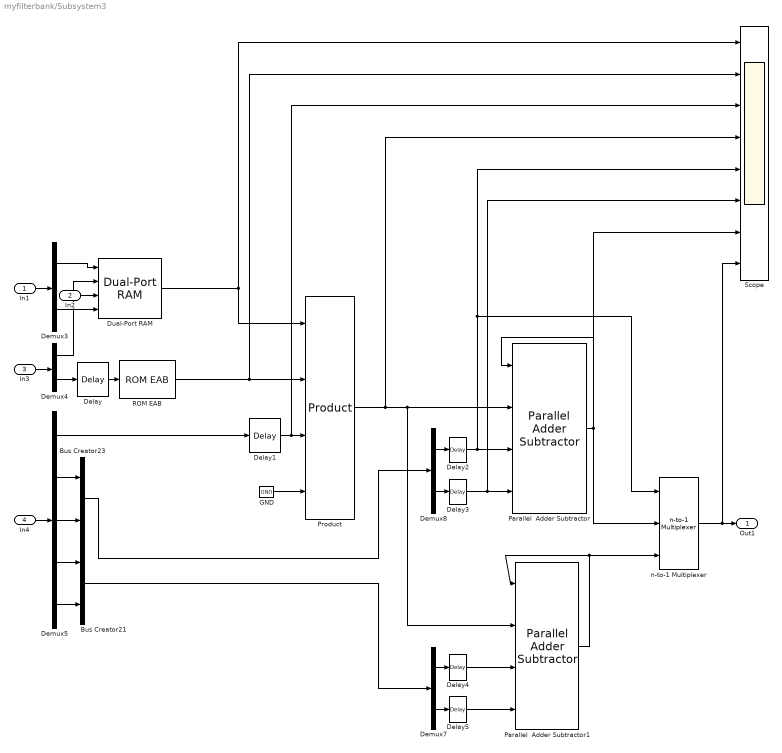
== system myfilterbank/Subsystem3 ==
  In1 : Inport  Port=1  LatchInput=off
  In2 : Inport  Port=2  LatchInput=off
  In3 : Inport  Port=3  LatchInput=off
  In4 : Inport  Port=4  LatchInput=off
  Bus Creator21 : BusCreator  Inputs=2
  Bus Creator23 : BusCreator  Inputs=2
  Delay : ALTELINK/Storage/Delay  depth=1  clken=off  MaskValue=1
  Delay1 : ALTELINK/Storage/Delay  depth=2  clken=off  MaskValue=1
  Delay{2..5} (4 alike) : ALTELINK/Storage/Delay  depth=3  clken=off  MaskValue=1
  Demux{3..4,7..8} (4 alike) : Demux  Outputs=2  BusSelectionMode=off
  Demux5 : Demux  Outputs=5  BusSelectionMode=off
  Dual-Port RAM : ALTELINK/Storage/Dual-Port RAM  bwaddr=9  MaskValue=1
  GND : ALTELINK/Bus Manipulation/GND
  Parallel  Adder Subtractor : ALTELINK/Arithmetic/Parallel  Adder Subtractor  Inputs=2  direction=++  pipeline=on  clken=on  MaskValue=1
  Parallel  Adder Subtractor1 : ALTELINK/Arithmetic/Parallel  Adder Subtractor  Inputs=2  direction=++  pipeline=on  clken=on  MaskValue=1
  Product : ALTELINK/Arithmetic/Product  pipeline=1  lpm=off  eab=off  clken=on  MaskValue=1
  ROM EAB : ALTELINK/Storage/ROM EAB  BusType=Signed Integer  bwl=14  bwr=0  bwaddr=9  Inputs=onlyone.hex  MaskValue=1
  Scope : Scope  NumInputPorts=8
      settings: TimeRange=auto  YMin=-5~-5~-5~-5~-5~-5~-5~-5  YMax=5~5~5~5~5~5~5~5  SaveToWorkspace=off  SaveName=ScopeData  LimitDataPoints=on  MaxDataPoints=20000
  n-to-1 Multiplexer : ALTELINK/Gates/n-to-1 Multiplexer  Inputs=2  BusType=off
  Out1 : Outport  Port=1
  wires:
  Dual-Port RAM/1 -> Product/1, Scope/1
  ROM EAB/1 -> Product/2, Scope/2
  Product/1 -> Parallel  Adder Subtractor/2, Parallel  Adder Subtractor1/2, Scope/4
  Parallel  Adder Subtractor1/1 -> Parallel  Adder Subtractor1/1, n-to-1 Multiplexer/3
  Parallel  Adder Subtractor/1 -> Parallel  Adder Subtractor/1, Scope/7, n-to-1 Multiplexer/2
  Delay/1 -> ROM EAB/1
  GND/1 -> Product/4
  Demux3/2 -> Dual-Port RAM/4
  Demux3/1 -> Dual-Port RAM/1
  Demux4/1 -> Dual-Port RAM/2
  Demux4/2 -> Delay/1
  Demux5/1 -> Delay1/1
  Delay1/1 -> Product/3, Scope/3
  Demux7/2 -> Delay5/1
  Demux7/1 -> Delay4/1
  Demux8/2 -> Delay3/1
  Demux8/1 -> Delay2/1
  Demux5/5 -> Bus Creator21/2
  Demux5/4 -> Bus Creator21/1
  Demux5/3 -> Bus Creator23/2
  Demux5/2 -> Bus Creator23/1
  Bus Creator21/1 -> Demux7/1
  Bus Creator23/1 -> Demux8/1
  Delay2/1 -> Parallel  Adder Subtractor/3, Scope/5, n-to-1 Multiplexer/1
  Delay3/1 -> Parallel  Adder Subtractor/4, Scope/6
  Delay4/1 -> Parallel  Adder Subtractor1/3
  Delay5/1 -> Parallel  Adder Subtractor1/4
  n-to-1 Multiplexer/1 -> Scope/8, Out1/1
  In1/1 -> Demux3/1
  In2/1 -> Dual-Port RAM/3
  In3/1 -> Demux4/1
  In4/1 -> Demux5/1

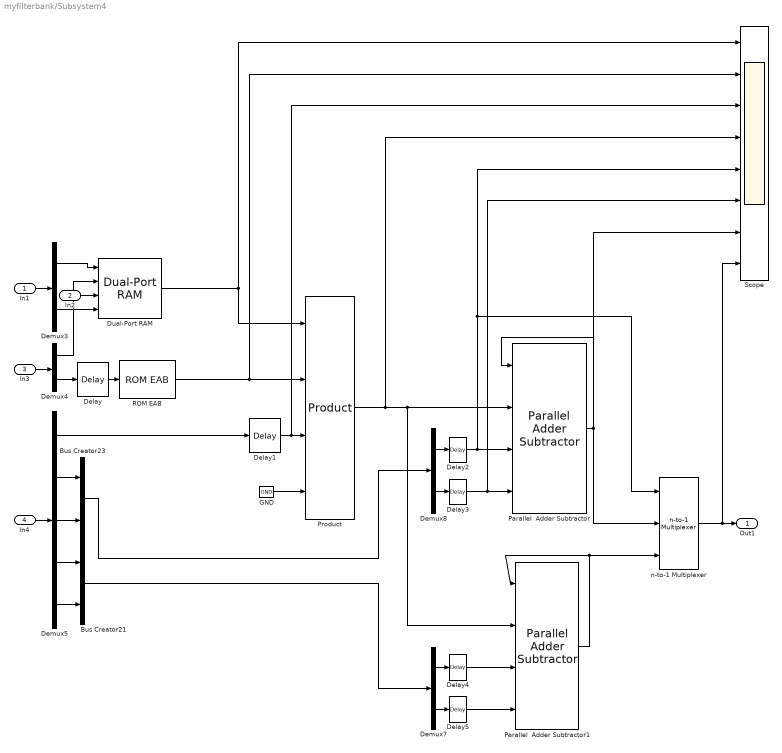
== system myfilterbank/Subsystem4 ==
  In1 : Inport  Port=1  LatchInput=off
  In2 : Inport  Port=2  LatchInput=off
  In3 : Inport  Port=3  LatchInput=off
  In4 : Inport  Port=4  LatchInput=off
  Bus Creator21 : BusCreator  Inputs=2
  Bus Creator23 : BusCreator  Inputs=2
  Delay : ALTELINK/Storage/Delay  depth=1  clken=off  MaskValue=1
  Delay1 : ALTELINK/Storage/Delay  depth=2  clken=off  MaskValue=1
  Delay{2..5} (4 alike) : ALTELINK/Storage/Delay  depth=3  clken=off  MaskValue=1
  Demux{3..4,7..8} (4 alike) : Demux  Outputs=2  BusSelectionMode=off
  Demux5 : Demux  Outputs=5  BusSelectionMode=off
  Dual-Port RAM : ALTELINK/Storage/Dual-Port RAM  bwaddr=9  MaskValue=1
  GND : ALTELINK/Bus Manipulation/GND
  Parallel  Adder Subtractor : ALTELINK/Arithmetic/Parallel  Adder Subtractor  Inputs=2  direction=++  pipeline=on  clken=on  MaskValue=1
  Parallel  Adder Subtractor1 : ALTELINK/Arithmetic/Parallel  Adder Subtractor  Inputs=2  direction=++  pipeline=on  clken=on  MaskValue=1
  Product : ALTELINK/Arithmetic/Product  pipeline=1  lpm=off  eab=off  clken=on  MaskValue=1
  ROM EAB : ALTELINK/Storage/ROM EAB  BusType=Signed Integer  bwl=14  bwr=0  bwaddr=9  Inputs=onlyone.hex  MaskValue=1
  Scope : Scope  NumInputPorts=8
      settings: TimeRange=auto  YMin=-5~-5~-5~-5~-5~-5~-5~-5  YMax=5~5~5~5~5~5~5~5  SaveToWorkspace=off  SaveName=ScopeData  LimitDataPoints=on  MaxDataPoints=20000
  n-to-1 Multiplexer : ALTELINK/Gates/n-to-1 Multiplexer  Inputs=2  BusType=off
  Out1 : Outport  Port=1
  wires:
  Dual-Port RAM/1 -> Product/1, Scope/1
  ROM EAB/1 -> Product/2, Scope/2
  Product/1 -> Parallel  Adder Subtractor/2, Parallel  Adder Subtractor1/2, Scope/4
  Parallel  Adder Subtractor1/1 -> Parallel  Adder Subtractor1/1, n-to-1 Multiplexer/3
  Parallel  Adder Subtractor/1 -> Parallel  Adder Subtractor/1, Scope/7, n-to-1 Multiplexer/2
  Delay/1 -> ROM EAB/1
  GND/1 -> Product/4
  Demux3/2 -> Dual-Port RAM/4
  Demux3/1 -> Dual-Port RAM/1
  Demux4/1 -> Dual-Port RAM/2
  Demux4/2 -> Delay/1
  Demux5/1 -> Delay1/1
  Delay1/1 -> Product/3, Scope/3
  Demux7/2 -> Delay5/1
  Demux7/1 -> Delay4/1
  Demux8/2 -> Delay3/1
  Demux8/1 -> Delay2/1
  Demux5/5 -> Bus Creator21/2
  Demux5/4 -> Bus Creator21/1
  Demux5/3 -> Bus Creator23/2
  Demux5/2 -> Bus Creator23/1
  Bus Creator21/1 -> Demux7/1
  Bus Creator23/1 -> Demux8/1
  Delay2/1 -> Parallel  Adder Subtractor/3, Scope/5, n-to-1 Multiplexer/1
  Delay3/1 -> Parallel  Adder Subtractor/4, Scope/6
  Delay4/1 -> Parallel  Adder Subtractor1/3
  Delay5/1 -> Parallel  Adder Subtractor1/4
  n-to-1 Multiplexer/1 -> Scope/8, Out1/1
  In1/1 -> Demux3/1
  In2/1 -> Dual-Port RAM/3
  In3/1 -> Demux4/1
  In4/1 -> Demux5/1

== system myfilterbank/Subsystem5 ==
  In1 : Inport  Port=1  LatchInput=off
  In2 : Inport  Port=2  LatchInput=off
  In3 : Inport  Port=3  LatchInput=off
  In4 : Inport  Port=4  LatchInput=off
  Bus Creator21 : BusCreator  Inputs=2
  Bus Creator23 : BusCreator  Inputs=2
  Delay : ALTELINK/Storage/Delay  depth=1  clken=off  MaskValue=1
  Delay1 : ALTELINK/Storage/Delay  depth=2  clken=off  MaskValue=1
  Delay{2..5} (4 alike) : ALTELINK/Storage/Delay  depth=3  clken=off  MaskValue=1
  Demux{3..4,7..8} (4 alike) : Demux  Outputs=2  BusSelectionMode=off
  Demux5 : Demux  Outputs=5  BusSelectionMode=off
  Dual-Port RAM : ALTELINK/Storage/Dual-Port RAM  bwaddr=9  MaskValue=1
  GND : ALTELINK/Bus Manipulation/GND
  Parallel  Adder Subtractor : ALTELINK/Arithmetic/Parallel  Adder Subtractor  Inputs=2  direction=++  pipeline=on  clken=on  MaskValue=1
  Parallel  Adder Subtractor1 : ALTELINK/Arithmetic/Parallel  Adder Subtractor  Inputs=2  direction=++  pipeline=on  clken=on  MaskValue=1
  Product : ALTELINK/Arithmetic/Product  pipeline=1  lpm=off  eab=off  clken=on  MaskValue=1
  ROM EAB : ALTELINK/Storage/ROM EAB  BusType=Signed Integer  bwl=14  bwr=0  bwaddr=9  Inputs=onlyone.hex  MaskValue=1
  Scope : Scope  NumInputPorts=8
      settings: TimeRange=auto  YMin=-5~-5~-5~-5~-5~-5~-5~-5  YMax=5~5~5~5~5~5~5~5  SaveToWorkspace=off  SaveName=ScopeData  LimitDataPoints=on  MaxDataPoints=20000
  n-to-1 Multiplexer : ALTELINK/Gates/n-to-1 Multiplexer  Inputs=2  BusType=off
  Out1 : Outport  Port=1
  wires:
  Dual-Port RAM/1 -> Product/1, Scope/1
  ROM EAB/1 -> Product/2, Scope/2
  Product/1 -> Parallel  Adder Subtractor/2, Parallel  Adder Subtractor1/2, Scope/4
  Parallel  Adder Subtractor1/1 -> Parallel  Adder Subtractor1/1, n-to-1 Multiplexer/3
  Parallel  Adder Subtractor/1 -> Parallel  Adder Subtractor/1, Scope/7, n-to-1 Multiplexer/2
  Delay/1 -> ROM EAB/1
  GND/1 -> Product/4
  Demux3/2 -> Dual-Port RAM/4
  Demux3/1 -> Dual-Port RAM/1
  Demux4/1 -> Dual-Port RAM/2
  Demux4/2 -> Delay/1
  Demux5/1 -> Delay1/1
  Delay1/1 -> Product/3, Scope/3
  Demux7/2 -> Delay5/1
  Demux7/1 -> Delay4/1
  Demux8/2 -> Delay3/1
  Demux8/1 -> Delay2/1
  Demux5/5 -> Bus Creator21/2
  Demux5/4 -> Bus Creator21/1
  Demux5/3 -> Bus Creator23/2
  Demux5/2 -> Bus Creator23/1
  Bus Creator21/1 -> Demux7/1
  Bus Creator23/1 -> Demux8/1
  Delay2/1 -> Parallel  Adder Subtractor/3, Scope/5, n-to-1 Multiplexer/1
  Delay3/1 -> Parallel  Adder Subtractor/4, Scope/6
  Delay4/1 -> Parallel  Adder Subtractor1/3
  Delay5/1 -> Parallel  Adder Subtractor1/4
  n-to-1 Multiplexer/1 -> Scope/8, Out1/1
  In1/1 -> Demux3/1
  In2/1 -> Dual-Port RAM/3
  In3/1 -> Demux4/1
  In4/1 -> Demux5/1

== system myfilterbank/Subsystem6 ==
  In1 : Inport  Port=1  LatchInput=off
  In2 : Inport  Port=2  LatchInput=off
  In3 : Inport  Port=3  LatchInput=off
  In4 : Inport  Port=4  LatchInput=off
  Bus Creator21 : BusCreator  Inputs=2
  Bus Creator23 : BusCreator  Inputs=2
  Delay : ALTELINK/Storage/Delay  depth=1  clken=off  MaskValue=1
  Delay1 : ALTELINK/Storage/Delay  depth=2  clken=off  MaskValue=1
  Delay{2..5} (4 alike) : ALTELINK/Storage/Delay  depth=3  clken=off  MaskValue=1
  Demux{3..4,7..8} (4 alike) : Demux  Outputs=2  BusSelectionMode=off
  Demux5 : Demux  Outputs=5  BusSelectionMode=off
  Dual-Port RAM : ALTELINK/Storage/Dual-Port RAM  bwaddr=9  MaskValue=1
  GND : ALTELINK/Bus Manipulation/GND
  Parallel  Adder Subtractor : ALTELINK/Arithmetic/Parallel  Adder Subtractor  Inputs=2  direction=++  pipeline=on  clken=on  MaskValue=1
  Parallel  Adder Subtractor1 : ALTELINK/Arithmetic/Parallel  Adder Subtractor  Inputs=2  direction=++  pipeline=on  clken=on  MaskValue=1
  Product : ALTELINK/Arithmetic/Product  pipeline=1  lpm=off  eab=off  clken=on  MaskValue=1
  ROM EAB : ALTELINK/Storage/ROM EAB  BusType=Signed Integer  bwl=14  bwr=0  bwaddr=9  Inputs=onlyone.hex  MaskValue=1
  Scope : Scope  NumInputPorts=8
      settings: TimeRange=auto  YMin=-5~-5~-5~-5~-5~-5~-5~-5  YMax=5~5~5~5~5~5~5~5  SaveToWorkspace=off  SaveName=ScopeData  LimitDataPoints=on  MaxDataPoints=20000
  n-to-1 Multiplexer : ALTELINK/Gates/n-to-1 Multiplexer  Inputs=2  BusType=off
  Out1 : Outport  Port=1
  wires:
  Dual-Port RAM/1 -> Product/1, Scope/1
  ROM EAB/1 -> Product/2, Scope/2
  Product/1 -> Parallel  Adder Subtractor/2, Parallel  Adder Subtractor1/2, Scope/4
  Parallel  Adder Subtractor1/1 -> Parallel  Adder Subtractor1/1, n-to-1 Multiplexer/3
  Parallel  Adder Subtractor/1 -> Parallel  Adder Subtractor/1, Scope/7, n-to-1 Multiplexer/2
  Delay/1 -> ROM EAB/1
  GND/1 -> Product/4
  Demux3/2 -> Dual-Port RAM/4
  Demux3/1 -> Dual-Port RAM/1
  Demux4/1 -> Dual-Port RAM/2
  Demux4/2 -> Delay/1
  Demux5/1 -> Delay1/1
  Delay1/1 -> Product/3, Scope/3
  Demux7/2 -> Delay5/1
  Demux7/1 -> Delay4/1
  Demux8/2 -> Delay3/1
  Demux8/1 -> Delay2/1
  Demux5/5 -> Bus Creator21/2
  Demux5/4 -> Bus Creator21/1
  Demux5/3 -> Bus Creator23/2
  Demux5/2 -> Bus Creator23/1
  Bus Creator21/1 -> Demux7/1
  Bus Creator23/1 -> Demux8/1
  Delay2/1 -> Parallel  Adder Subtractor/3, Scope/5, n-to-1 Multiplexer/1
  Delay3/1 -> Parallel  Adder Subtractor/4, Scope/6
  Delay4/1 -> Parallel  Adder Subtractor1/3
  Delay5/1 -> Parallel  Adder Subtractor1/4
  n-to-1 Multiplexer/1 -> Scope/8, Out1/1
  In1/1 -> Demux3/1
  In2/1 -> Dual-Port RAM/3
  In3/1 -> Demux4/1
  In4/1 -> Demux5/1

== system myfilterbank/Subsystem7 ==
  In1 : Inport  Port=1  LatchInput=off
  In2 : Inport  Port=2  LatchInput=off
  In3 : Inport  Port=3  LatchInput=off
  In4 : Inport  Port=4  LatchInput=off
  Bus Creator21 : BusCreator  Inputs=2
  Bus Creator23 : BusCreator  Inputs=2
  Delay : ALTELINK/Storage/Delay  depth=1  clken=off  MaskValue=1
  Delay1 : ALTELINK/Storage/Delay  depth=2  clken=off  MaskValue=1
  Delay{2..5} (4 alike) : ALTELINK/Storage/Delay  depth=3  clken=off  MaskValue=1
  Demux{3..4,7..8} (4 alike) : Demux  Outputs=2  BusSelectionMode=off
  Demux5 : Demux  Outputs=5  BusSelectionMode=off
  Dual-Port RAM : ALTELINK/Storage/Dual-Port RAM  bwaddr=9  MaskValue=1
  GND : ALTELINK/Bus Manipulation/GND
  Parallel  Adder Subtractor : ALTELINK/Arithmetic/Parallel  Adder Subtractor  Inputs=2  direction=++  pipeline=on  clken=on  MaskValue=1
  Parallel  Adder Subtractor1 : ALTELINK/Arithmetic/Parallel  Adder Subtractor  Inputs=2  direction=++  pipeline=on  clken=on  MaskValue=1
  Product : ALTELINK/Arithmetic/Product  pipeline=1  lpm=off  eab=off  clken=on  MaskValue=1
  ROM EAB : ALTELINK/Storage/ROM EAB  BusType=Signed Integer  bwl=14  bwr=0  bwaddr=9  Inputs=onlyone.hex  MaskValue=1
  Scope : Scope  NumInputPorts=8
      settings: TimeRange=auto  YMin=-5~-5~-5~-5~-5~-5~-5~-5  YMax=5~5~5~5~5~5~5~5  SaveToWorkspace=off  SaveName=ScopeData  LimitDataPoints=on  MaxDataPoints=20000
  n-to-1 Multiplexer : ALTELINK/Gates/n-to-1 Multiplexer  Inputs=2  BusType=off
  Out1 : Outport  Port=1
  wires:
  Dual-Port RAM/1 -> Product/1, Scope/1
  ROM EAB/1 -> Product/2, Scope/2
  Product/1 -> Parallel  Adder Subtractor/2, Parallel  Adder Subtractor1/2, Scope/4
  Parallel  Adder Subtractor1/1 -> Parallel  Adder Subtractor1/1, n-to-1 Multiplexer/3
  Parallel  Adder Subtractor/1 -> Parallel  Adder Subtractor/1, Scope/7, n-to-1 Multiplexer/2
  Delay/1 -> ROM EAB/1
  GND/1 -> Product/4
  Demux3/2 -> Dual-Port RAM/4
  Demux3/1 -> Dual-Port RAM/1
  Demux4/1 -> Dual-Port RAM/2
  Demux4/2 -> Delay/1
  Demux5/1 -> Delay1/1
  Delay1/1 -> Product/3, Scope/3
  Demux7/2 -> Delay5/1
  Demux7/1 -> Delay4/1
  Demux8/2 -> Delay3/1
  Demux8/1 -> Delay2/1
  Demux5/5 -> Bus Creator21/2
  Demux5/4 -> Bus Creator21/1
  Demux5/3 -> Bus Creator23/2
  Demux5/2 -> Bus Creator23/1
  Bus Creator21/1 -> Demux7/1
  Bus Creator23/1 -> Demux8/1
  Delay2/1 -> Parallel  Adder Subtractor/3, Scope/5, n-to-1 Multiplexer/1
  Delay3/1 -> Parallel  Adder Subtractor/4, Scope/6
  Delay4/1 -> Parallel  Adder Subtractor1/3
  Delay5/1 -> Parallel  Adder Subtractor1/4
  n-to-1 Multiplexer/1 -> Scope/8, Out1/1
  In1/1 -> Demux3/1
  In2/1 -> Dual-Port RAM/3
  In3/1 -> Demux4/1
  In4/1 -> Demux5/1

== system myfilterbank/Subsystem8 ==
  In1 : Inport  Port=1  LatchInput=off
  In2 : Inport  Port=2  LatchInput=off
  In3 : Inport  Port=3  LatchInput=off
  In4 : Inport  Port=4  LatchInput=off
  Bus Creator21 : BusCreator  Inputs=2
  Bus Creator23 : BusCreator  Inputs=2
  Delay : ALTELINK/Storage/Delay  depth=1  clken=off  MaskValue=1
  Delay1 : ALTELINK/Storage/Delay  depth=2  clken=off  MaskValue=1
  Delay{2..5} (4 alike) : ALTELINK/Storage/Delay  depth=3  clken=off  MaskValue=1
  Demux{3..4,7..8} (4 alike) : Demux  Outputs=2  BusSelectionMode=off
  Demux5 : Demux  Outputs=5  BusSelectionMode=off
  Dual-Port RAM : ALTELINK/Storage/Dual-Port RAM  bwaddr=9  MaskValue=1
  GND : ALTELINK/Bus Manipulation/GND
  Parallel  Adder Subtractor : ALTELINK/Arithmetic/Parallel  Adder Subtractor  Inputs=2  direction=++  pipeline=on  clken=on  MaskValue=1
  Parallel  Adder Subtractor1 : ALTELINK/Arithmetic/Parallel  Adder Subtractor  Inputs=2  direction=++  pipeline=on  clken=on  MaskValue=1
  Product : ALTELINK/Arithmetic/Product  pipeline=1  lpm=off  eab=off  clken=on  MaskValue=1
  ROM EAB : ALTELINK/Storage/ROM EAB  BusType=Signed Integer  bwl=14  bwr=0  bwaddr=9  Inputs=onlyone.hex  MaskValue=1
  Scope : Scope  NumInputPorts=8
      settings: TimeRange=auto  YMin=-5~-5~-5~-5~-5~-5~-5~-5  YMax=5~5~5~5~5~5~5~5  SaveToWorkspace=off  SaveName=ScopeData  LimitDataPoints=on  MaxDataPoints=20000
  n-to-1 Multiplexer : ALTELINK/Gates/n-to-1 Multiplexer  Inputs=2  BusType=off
  Out1 : Outport  Port=1
  wires:
  Dual-Port RAM/1 -> Product/1, Scope/1
  ROM EAB/1 -> Product/2, Scope/2
  Product/1 -> Parallel  Adder Subtractor/2, Parallel  Adder Subtractor1/2, Scope/4
  Parallel  Adder Subtractor1/1 -> Parallel  Adder Subtractor1/1, n-to-1 Multiplexer/3
  Parallel  Adder Subtractor/1 -> Parallel  Adder Subtractor/1, Scope/7, n-to-1 Multiplexer/2
  Delay/1 -> ROM EAB/1
  GND/1 -> Product/4
  Demux3/2 -> Dual-Port RAM/4
  Demux3/1 -> Dual-Port RAM/1
  Demux4/1 -> Dual-Port RAM/2
  Demux4/2 -> Delay/1
  Demux5/1 -> Delay1/1
  Delay1/1 -> Product/3, Scope/3
  Demux7/2 -> Delay5/1
  Demux7/1 -> Delay4/1
  Demux8/2 -> Delay3/1
  Demux8/1 -> Delay2/1
  Demux5/5 -> Bus Creator21/2
  Demux5/4 -> Bus Creator21/1
  Demux5/3 -> Bus Creator23/2
  Demux5/2 -> Bus Creator23/1
  Bus Creator21/1 -> Demux7/1
  Bus Creator23/1 -> Demux8/1
  Delay2/1 -> Parallel  Adder Subtractor/3, Scope/5, n-to-1 Multiplexer/1
  Delay3/1 -> Parallel  Adder Subtractor/4, Scope/6
  Delay4/1 -> Parallel  Adder Subtractor1/3
  Delay5/1 -> Parallel  Adder Subtractor1/4
  n-to-1 Multiplexer/1 -> Scope/8, Out1/1
  In1/1 -> Demux3/1
  In2/1 -> Dual-Port RAM/3
  In3/1 -> Demux4/1
  In4/1 -> Demux5/1

== system myfilterbank/Subsystem9 ==
  In1 : Inport  Port=1  LatchInput=off
  In2 : Inport  Port=2  LatchInput=off
  In3 : Inport  Port=3  LatchInput=off
  In4 : Inport  Port=4  LatchInput=off
  Bus Creator21 : BusCreator  Inputs=2
  Bus Creator23 : BusCreator  Inputs=2
  Delay : ALTELINK/Storage/Delay  depth=1  clken=off  MaskValue=1
  Delay1 : ALTELINK/Storage/Delay  depth=2  clken=off  MaskValue=1
  Delay{2..5} (4 alike) : ALTELINK/Storage/Delay  depth=3  clken=off  MaskValue=1
  Demux{3..4,7..8} (4 alike) : Demux  Outputs=2  BusSelectionMode=off
  Demux5 : Demux  Outputs=5  BusSelectionMode=off
  Dual-Port RAM : ALTELINK/Storage/Dual-Port RAM  bwaddr=9  MaskValue=1
  GND : ALTELINK/Bus Manipulation/GND
  Parallel  Adder Subtractor : ALTELINK/Arithmetic/Parallel  Adder Subtractor  Inputs=2  direction=++  pipeline=on  clken=on  MaskValue=1
  Parallel  Adder Subtractor1 : ALTELINK/Arithmetic/Parallel  Adder Subtractor  Inputs=2  direction=++  pipeline=on  clken=on  MaskValue=1
  Product : ALTELINK/Arithmetic/Product  pipeline=1  lpm=off  eab=off  clken=on  MaskValue=1
  ROM EAB : ALTELINK/Storage/ROM EAB  BusType=Signed Integer  bwl=14  bwr=0  bwaddr=9  Inputs=onlyone.hex  MaskValue=1
  Scope : Scope  NumInputPorts=8
      settings: TimeRange=auto  YMin=-5~-5~-5~-5~-5~-5~-5~-5  YMax=5~5~5~5~5~5~5~5  SaveToWorkspace=off  SaveName=ScopeData  LimitDataPoints=on  MaxDataPoints=20000
  n-to-1 Multiplexer : ALTELINK/Gates/n-to-1 Multiplexer  Inputs=2  BusType=off
  Out1 : Outport  Port=1
  wires:
  Dual-Port RAM/1 -> Product/1, Scope/1
  ROM EAB/1 -> Product/2, Scope/2
  Product/1 -> Parallel  Adder Subtractor/2, Parallel  Adder Subtractor1/2, Scope/4
  Parallel  Adder Subtractor1/1 -> Parallel  Adder Subtractor1/1, n-to-1 Multiplexer/3
  Parallel  Adder Subtractor/1 -> Parallel  Adder Subtractor/1, Scope/7, n-to-1 Multiplexer/2
  Delay/1 -> ROM EAB/1
  GND/1 -> Product/4
  Demux3/2 -> Dual-Port RAM/4
  Demux3/1 -> Dual-Port RAM/1
  Demux4/1 -> Dual-Port RAM/2
  Demux4/2 -> Delay/1
  Demux5/1 -> Delay1/1
  Delay1/1 -> Product/3, Scope/3
  Demux7/2 -> Delay5/1
  Demux7/1 -> Delay4/1
  Demux8/2 -> Delay3/1
  Demux8/1 -> Delay2/1
  Demux5/5 -> Bus Creator21/2
  Demux5/4 -> Bus Creator21/1
  Demux5/3 -> Bus Creator23/2
  Demux5/2 -> Bus Creator23/1
  Bus Creator21/1 -> Demux7/1
  Bus Creator23/1 -> Demux8/1
  Delay2/1 -> Parallel  Adder Subtractor/3, Scope/5, n-to-1 Multiplexer/1
  Delay3/1 -> Parallel  Adder Subtractor/4, Scope/6
  Delay4/1 -> Parallel  Adder Subtractor1/3
  Delay5/1 -> Parallel  Adder Subtractor1/4
  n-to-1 Multiplexer/1 -> Scope/8, Out1/1
  In1/1 -> Demux3/1
  In2/1 -> Dual-Port RAM/3
  In3/1 -> Demux4/1
  In4/1 -> Demux5/1
